simulink model "control_onoff"  (R2020b)
settings: Solver=VariableStepAuto  StartTime=0.0  StopTime=50  RelTol=1e-3
values from neighbouring files (symbols this model uses):
  C = 4    [control_on_off.m]
  R = 2    [control_on_off.m]
libraries: simulink x1
settings Model: Creator=carma  LastModifiedBy=carma
settings SolverCC: ZeroCrossAlgorithm=Adaptive
settings DebuggingCC: IgnoredZcDiagnostic=none

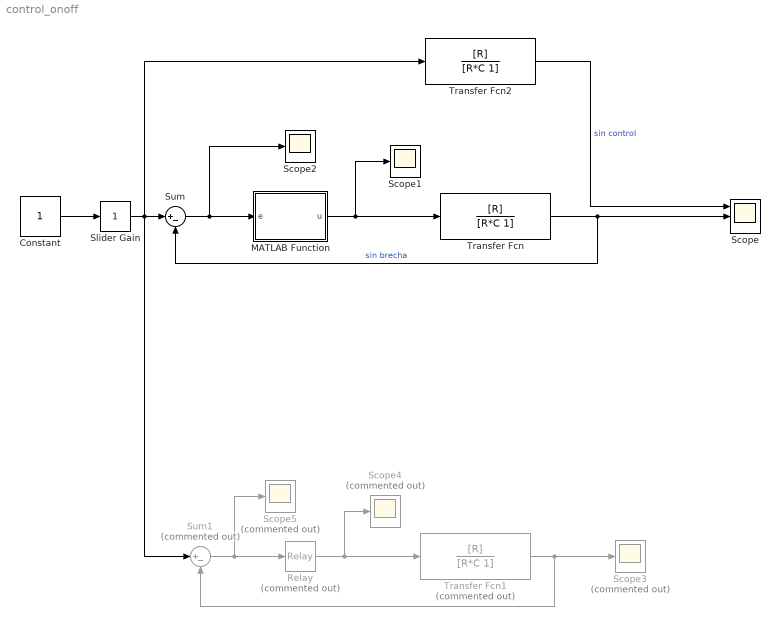
== system control_onoff ==
  Constant : Constant  VectorParams1D=off  SampleTime=-1
  MATLAB Function : MATLAB Function  TreatAsAtomicUnit=on
  Relay : Relay  Commented=on
  Scope : Scope  NumInputPorts=3
  Scope1 : Scope
  Scope2 : Scope
  Scope3 : Scope  Commented=on
  Scope4 : Scope  Commented=on
  Scope5 : Scope  Commented=on
  Slider Gain : simulink/Math Operations/Slider Gain  gain=1  low=0  high=2
  Sum : Sum  Inputs=|+-
  Sum1 : Sum  Commented=on  Inputs=|+-
  Transfer Fcn : TransferFcn  Numerator=[R]  Denominator=[R*C 1]
  Transfer Fcn1 : TransferFcn  Commented=on  Numerator=[R]  Denominator=[R*C 1]
  Transfer Fcn2 : TransferFcn  Numerator=[R]  Denominator=[R*C 1]
  wires:
  Transfer Fcn/1 -> Sum/2, Scope/2  "sin brecha"
  Sum/1 -> MATLAB Function/1(e), Scope2/1
  MATLAB Function/1(u) -> Scope1/1, Transfer Fcn/1
  Constant/1 -> Slider Gain/1
  Relay/1 -> Scope4/1, Transfer Fcn1/1
  Sum1/1 -> Scope5/1, Relay/1
  Transfer Fcn1/1 -> Sum1/2, Scope3/1
  Transfer Fcn2/1 -> Scope/1  "sin control"
  Slider Gain/1 -> Sum1/1, Transfer Fcn2/1, Sum/1

== matlab function control_onoff/MATLAB Function ==
  data: e input; u output
function u = fcn(e)
%SIN BRECHA DIFERENCIAL
if e >=0
    u = 1;
else
    u=0;
end
end
